simulink model "MBS_FlexibleBoom_Inverse_Dynamics"  (R2020b)
settings: Solver=ode23t  StartTime=0  StopTime=17  FixedStep=.00001  MaxStep=1e-3  RelTol=1e-3
model workspace: external: MATLAB File C:\GitHub\UiA_GreenCrane_TestBed\Simulation Models\Crane\Rigid - MBS model\param_MBS_FlexibleBoom_Inverse_Dynamics.m (data not in the file)
values from neighbouring files (symbols this model uses):
  d_eff_long = sqrt(2*J_sec_long*k_eff_long)    [param_MBS_FlexibleBoom_Inverse_Dynamics.m]
  d_eff_short = sqrt(2*J_sec_short*k_eff_short)    [param_MBS_FlexibleBoom_Inverse_Dynamics.m]
  DR = 1    [param_MBS_FlexibleBoom_Inverse_Dynamics.m]
  k_eff_long = E*I/I_sec_long    (= 3050381.94041)    [param_MBS_FlexibleBoom_Inverse_Dynamics.m]
  k_eff_short = E*I/I_sec_short    (= 13451432.5427)    [param_MBS_FlexibleBoom_Inverse_Dynamics.m]
  KR = 1    [param_MBS_FlexibleBoom_Inverse_Dynamics.m]
  v_cyl_0 = 0.0    (= 0)    [param_MBS_FlexibleBoom_Inverse_Dynamics.m]
  x_cyl_0 = 0.05    [param_MBS_FlexibleBoom_Inverse_Dynamics.m]
undefined symbols (not defined in the file or in its folder): smiData, X, Y, Z
libraries: sm_lib x190, nesl_utility x26
(part 1 of 5)
settings Model: Creator=Zygis  LastModifiedBy=danielh
settings SolverCC: ZeroCrossAlgorithm=Adaptive
settings DataIOCC: ExternalInput=getinputstruct(report1)  InitialState=getstatestruct(report1)  ReturnWorkspaceOutputs=off  Refine=2
settings DebuggingCC: IgnoredZcDiagnostic=none  UniqueDataStoreMsg=error  UnderSpecifiedDimensionMsg=warning  ArithmeticOperatorsInVariantConditions=warning
settings HardwareCC: TargetBitPerPointer=64  TargetBitPerSizeT=64  TargetBitPerPtrDiffT=64  TargetLongLongMode=on  TargetIntDivRoundTo=Zero  TargetEndianess=LittleEndian  TargetWordSize=64  TargetHWDeviceType=MATLAB Host  ProdEqTarget=off
settings SFSimCC: SimUseLocalCustomCode=off  CustomCodeUndefinedFunction=UseInterfaceOnly
settings RTWCC: Description=Rapid Simulation Target  SystemTargetFile=rsim.tlc  TemplateMakefile=rsim_default_tmf  GenerateReport=on  RTWUseLocalCustomCode=off
settings RSimTargetCC: TargetLangStandard=C99 (ISO)
settings DiagnosticsConfigSet: SimMechanicsJointTargetOverSpecification=warning

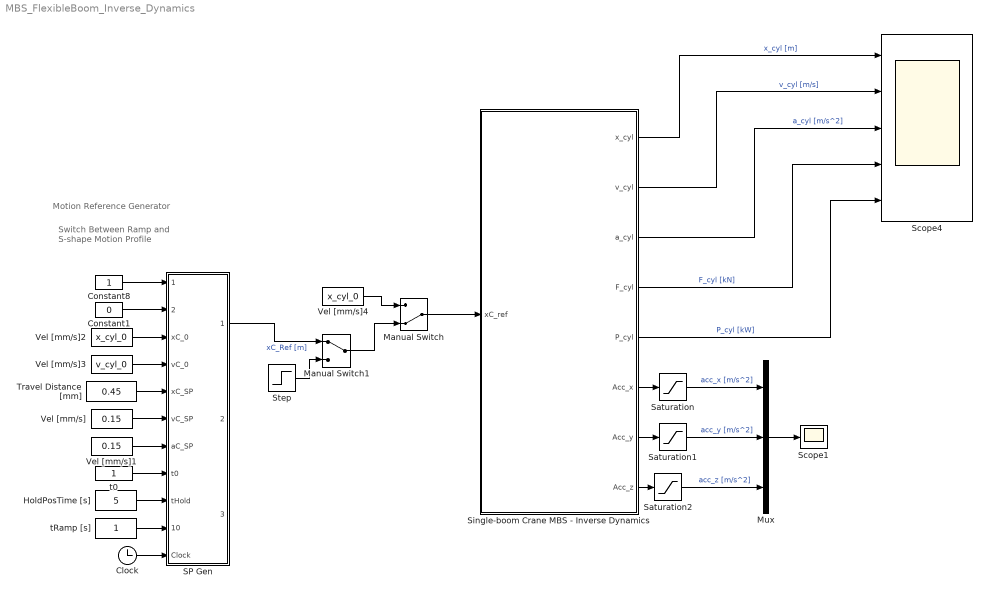
== system MBS_FlexibleBoom_Inverse_Dynamics ==
  note: Motion Reference Generator
  note: Switch Between
      | Ramp and S-shape
      | Motion Profile
  Clock : Clock
  Constant1 : Constant  Value=0  OutDataTypeStr=boolean
  Constant8 : Constant  OutDataTypeStr=boolean
  HoldPosTime [s] : Constant  Value=5
  Manual Switch : ManualSwitch  CurrentSetting=0
  Manual Switch1 : ManualSwitch
  Mux : Mux  Inputs=3
  SP Gen : Subsystem
  Saturation : Saturate  UpperLimit=2  LowerLimit=-2
  Saturation1 : Saturate  UpperLimit=2  LowerLimit=-2
  Saturation2 : Saturate  UpperLimit=2  LowerLimit=-2
  Scope1 : Scope
  Scope4 : Scope  NumInputPorts=5
  Single-boom Crane MBS - Inverse Dynamics : Subsystem  VariantControl=Flexible_model
  Step : Step  Before=x_cyl_0  After=0.1  SampleTime=0
  Travel Distance [mm] : Constant  Value=0.45
  Vel [mm/s] : Constant  Value=0.15
  Vel [mm/s]1 : Constant  Value=0.15
  Vel [mm/s]2 : Constant  Value=x_cyl_0
  Vel [mm/s]3 : Constant  Value=v_cyl_0
  Vel [mm/s]4 : Constant  Value=x_cyl_0
  t0 : Constant
  tRamp [s] : Constant
  wires:
  Single-boom Crane MBS - Inverse Dynamics/1(x_cyl) -> Scope4/1  "x_cyl [m]"
  Single-boom Crane MBS - Inverse Dynamics/2(v_cyl) -> Scope4/2  "v_cyl [m/s]"
  Manual Switch/1 -> Single-boom Crane MBS - Inverse Dynamics/1(xC_ref)
  Single-boom Crane MBS - Inverse Dynamics/3(a_cyl) -> Scope4/3  "a_cyl [m/s^2]"
  Single-boom Crane MBS - Inverse Dynamics/4(F_cyl) -> Scope4/4  "F_cyl [kN]"
  Vel [mm/s]3/1 -> SP Gen/4(vC_0)
  t0/1 -> SP Gen/8(t0)
  Constant8/1 -> SP Gen/1(Enable)
  Clock/1 -> SP Gen/11(Clock)
  Vel [mm/s]2/1 -> SP Gen/3(xC_0)
  Vel [mm/s]/1 -> SP Gen/6(vC_SP)
  Constant1/1 -> SP Gen/2(S-shape On)
  Travel Distance [mm]/1 -> SP Gen/5(xC_SP)
  tRamp [s]/1 -> SP Gen/10(tRamp)
  HoldPosTime [s]/1 -> SP Gen/9(tHold)
  Vel [mm/s]1/1 -> SP Gen/7(aC_SP)
  SP Gen/1(xC_ref) -> Manual Switch1/1  "xC_Ref [m]"
  Single-boom Crane MBS - Inverse Dynamics/5(P_cyl) -> Scope4/5  "P_cyl [kW]"
  Vel [mm/s]4/1 -> Manual Switch/1
  Step/1 -> Manual Switch1/2
  Manual Switch1/1 -> Manual Switch/2
  Single-boom Crane MBS - Inverse Dynamics/6(Acc_x) -> Saturation/1
  Single-boom Crane MBS - Inverse Dynamics/7(Acc_y) -> Saturation1/1
  Single-boom Crane MBS - Inverse Dynamics/8(Acc_z) -> Saturation2/1
  Mux/1 -> Scope1/1
  Saturation/1 -> Mux/1  "acc_x [m/s^2]"
  Saturation1/1 -> Mux/2  "acc_y [m/s^2]"
  Saturation2/1 -> Mux/3  "acc_z [m/s^2]"

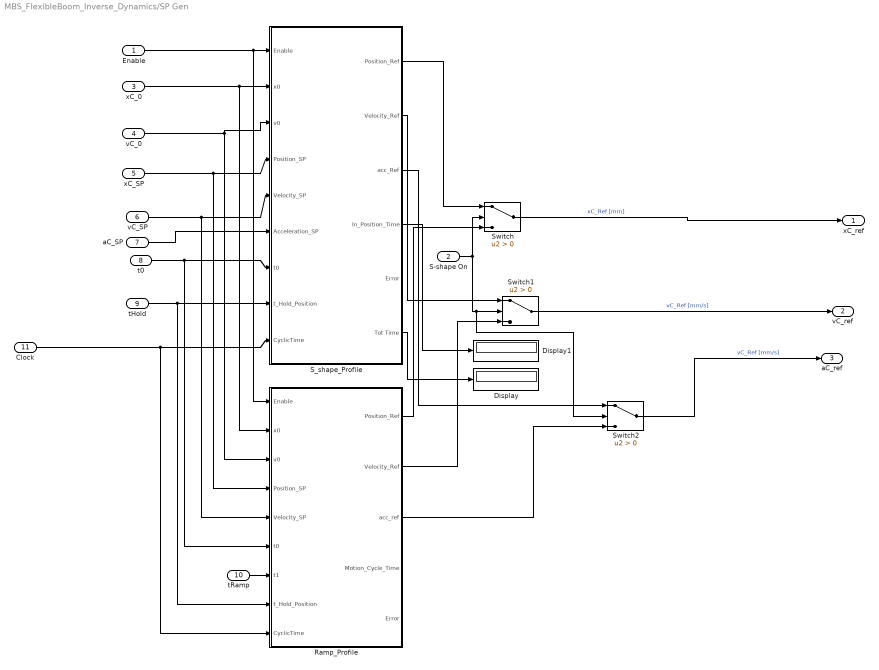
== system MBS_FlexibleBoom_Inverse_Dynamics/SP Gen ==
  Enable : Inport
  S-shape On : Inport  Port=2
  xC_0 : Inport  Port=3
  vC_0 : Inport  Port=4
  xC_SP : Inport  Port=5
  vC_SP : Inport  Port=6
  aC_SP : Inport  Port=7
  t0 : Inport  Port=8
  tHold : Inport  Port=9
  tRamp : Inport  Port=10
  Clock : Inport  Port=11
  Display : Display
  Display1 : Display
  Ramp_Profile : Subsystem  TreatAsAtomicUnit=on  VariantControl=Ramp_Profile
  S_shape_Profile : Subsystem  VariantControl=S_shape_Profile
  Switch : Switch  Criteria=u2 > Threshold
  Switch1 : Switch  Criteria=u2 > Threshold
  Switch2 : Switch  Criteria=u2 > Threshold
  xC_ref : Outport  VectorParamsAs1DForOutWhenUnconnected=off
  vC_ref : Outport  Port=2  VectorParamsAs1DForOutWhenUnconnected=off
  aC_ref : Outport  Port=3  VectorParamsAs1DForOutWhenUnconnected=off
  wires:
  t0/1 -> Ramp_Profile/6(t0), S_shape_Profile/7(t0)
  vC_SP/1 -> Ramp_Profile/5(Velocity_SP), S_shape_Profile/5(Velocity_SP)
  xC_0/1 -> Ramp_Profile/2(x0), S_shape_Profile/2(x0)
  xC_SP/1 -> Ramp_Profile/4(Position_SP), S_shape_Profile/4(Position_SP)
  Enable/1 -> Ramp_Profile/1(Enable), S_shape_Profile/1(Enable)
  tHold/1 -> Ramp_Profile/8(t_Hold_Position), S_shape_Profile/8(t_Hold_Position)
  S_shape_Profile/1(Position_Ref) -> Switch/1
  Ramp_Profile/1(Position_Ref) -> Switch/3
  S_shape_Profile/2(Velocity_Ref) -> Switch1/1
  S-shape On/1 -> Switch/2, Switch2/2, Switch1/2
  tRamp/1 -> Ramp_Profile/7(t1)
  S_shape_Profile/6(Tot Time) -> Display/1
  S_shape_Profile/4(" In_Position_Time") -> Display1/1
  vC_0/1 -> S_shape_Profile/3(v0), Ramp_Profile/3(v0)
  aC_SP/1 -> S_shape_Profile/6(Acceleration_SP)
  Clock/1 -> Ramp_Profile/9(CyclicTime), S_shape_Profile/9(CyclicTime)
  Switch/1 -> xC_ref/1  "xC_Ref [mm]"
  Switch1/1 -> vC_ref/1  "vC_Ref [mm/s]"
  Ramp_Profile/2(Velocity_Ref) -> Switch1/3
  Switch2/1 -> aC_ref/1  "vC_Ref [mm/s]"
  S_shape_Profile/3(acc_Ref) -> Switch2/1
  Ramp_Profile/3(acc_ref) -> Switch2/3

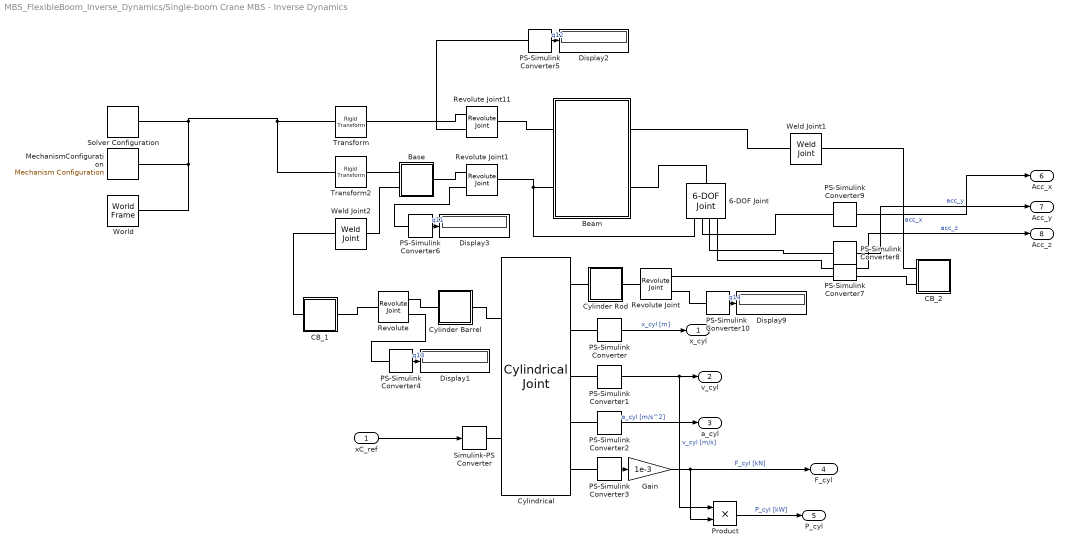
== system MBS_FlexibleBoom_Inverse_Dynamics/Single-boom Crane MBS - Inverse Dynamics ==
  xC_ref : Inport
  6-DOF Joint : sm_lib/Joints/6-DOF Joint  JointMode=Normal  SenseConstraintForce=off  SenseConstraintForceX=off  SenseConstraintForceY=off  SenseConstraintForceZ=off  SenseConstraintTorque=off  SenseConstraintTorqueX=off  SenseConstraintTorqueY=off  SenseConstraintTorqueZ=off  SenseTotalForce=off  SenseTotalForceX=off  SenseTotalForceY=off  SenseTotalForceZ=off  SenseTotalTorque=off  SenseTotalTorqueX=off  SenseTotalTorqueY=off  SenseTotalTorqueZ=off  CompositeWrenchDir=FollowerOnBase  CompositeWrenchFrame=BaseFrame  PxEquilibriumPosition=0  PxEquilibriumPositionUnits=m  PxSpringStiffness=0  PxSpringStiffnessUnits=N/m  PxDampingCoefficient=0  PxDampingCoefficientUnits=N/(m/s)  PxTorqueActuationMode=NoTorque  PxMotionActuationMode=ComputedMotion  PxSensePosition=off  PxSenseVelocity=off  PxSenseAcceleration=on  PxSenseTorqueForce=off  PxSenseLowerLimitTorqueForce=off  PxSenseUpperLimitTorqueForce=off  PxLowerLimitSpecify=off  PxLowerLimitBound=-1  PxLowerLimitBoundUnits=m  PxLowerLimitStiffness=1e6  PxLowerLimitStiffnessUnits=N/m  PxLowerLimitDamping=1e3  PxLowerLimitDampingUnits=N/(m/s)  PxLowerLimitTransitionRegionWidth=1e-4  PxLowerLimitTransitionRegionWidthUnits=m  PxUpperLimitSpecify=off  PxUpperLimitBound=1  PxUpperLimitBoundUnits=m  PxUpperLimitStiffness=1e6  PxUpperLimitStiffnessUnits=N/m  PxUpperLimitDamping=1e3  PxUpperLimitDampingUnits=N/(m/s)  PxUpperLimitTransitionRegionWidth=1e-4  PxUpperLimitTransitionRegionWidthUnits=m  PxPositionTargetSpecify=off  PxPositionTargetPriority=High  PxPositionTargetValue=0  PxPositionTargetValueUnits=m  PxVelocityTargetSpecify=off  PxVelocityTargetPriority=High  PxVelocityTargetValue=0  PxVelocityTargetValueUnits=m/s  PyEquilibriumPosition=0  PyEquilibriumPositionUnits=m  PySpringStiffness=0  PySpringStiffnessUnits=N/m  PyDampingCoefficient=0  PyDampingCoefficientUnits=N/(m/s)  PyTorqueActuationMode=NoTorque  PyMotionActuationMode=ComputedMotion  PySensePosition=off  PySenseVelocity=off  PySenseAcceleration=on  PySenseTorqueForce=off  PySenseLowerLimitTorqueForce=off  PySenseUpperLimitTorqueForce=off  PyLowerLimitSpecify=off  PyLowerLimitBound=-1  PyLowerLimitBoundUnits=m  PyLowerLimitStiffness=1e6  PyLowerLimitStiffnessUnits=N/m  PyLowerLimitDamping=1e3  PyLowerLimitDampingUnits=N/(m/s)  PyLowerLimitTransitionRegionWidth=1e-4  PyLowerLimitTransitionRegionWidthUnits=m  PyUpperLimitSpecify=off  PyUpperLimitBound=1  PyUpperLimitBoundUnits=m  PyUpperLimitStiffness=1e6  PyUpperLimitStiffnessUnits=N/m  PyUpperLimitDamping=1e3  PyUpperLimitDampingUnits=N/(m/s)  PyUpperLimitTransitionRegionWidth=1e-4  PyUpperLimitTransitionRegionWidthUnits=m  PyPositionTargetSpecify=off  PyPositionTargetPriority=High  PyPositionTargetValue=0  PyPositionTargetValueUnits=m  PyVelocityTargetSpecify=off  PyVelocityTargetPriority=High  PyVelocityTargetValue=0  PyVelocityTargetValueUnits=m/s  PzEquilibriumPosition=0  PzEquilibriumPositionUnits=m  PzSpringStiffness=0  PzSpringStiffnessUnits=N/m  PzDampingCoefficient=0  PzDampingCoefficientUnits=N/(m/s)  PzTorqueActuationMode=NoTorque  PzMotionActuationMode=ComputedMotion  PzSensePosition=off  PzSenseVelocity=off  PzSenseAcceleration=on  PzSenseTorqueForce=off  PzSenseLowerLimitTorqueForce=off  PzSenseUpperLimitTorqueForce=off  PzLowerLimitSpecify=off  PzLowerLimitBound=-1  PzLowerLimitBoundUnits=m  PzLowerLimitStiffness=1e6  PzLowerLimitStiffnessUnits=N/m  PzLowerLimitDamping=1e3  PzLowerLimitDampingUnits=N/(m/s)  PzLowerLimitTransitionRegionWidth=1e-4  PzLowerLimitTransitionRegionWidthUnits=m  PzUpperLimitSpecify=off  PzUpperLimitBound=1  PzUpperLimitBoundUnits=m  PzUpperLimitStiffness=1e6  PzUpperLimitStiffnessUnits=N/m  PzUpperLimitDamping=1e3  PzUpperLimitDampingUnits=N/(m/s)  PzUpperLimitTransitionRegionWidth=1e-4  PzUpperLimitTransitionRegionWidthUnits=m  PzPositionTargetSpecify=off  PzPositionTargetPriority=High  PzPositionTargetValue=0  PzPositionTargetValueUnits=m  PzVelocityTargetSpecify=off  PzVelocityTargetPriority=High  PzVelocityTargetValue=0  PzVelocityTargetValueUnits=m/s  SphDefPosRotationMethod=None  SphDefPosRotationAngleUnits=deg  SphDefPosRotationStandardAxis=+Z  SphDefPosRotationAngle=0.0  SphDefPosRotationArbitraryAxis=[0 0 1]  SphDefPosFollAlignAxisA=+X  SphDefPosBaseAlignAxisA=+Y  SphDefPosFollAlignAxisB=+Y  SphDefPosBaseAlignAxisB=+Z  SphDefPosRotationSequenceAxes=FollowerAxes  SphDefPosRotationSequence=XYX  SphDefPosRotationSequenceAngles=[0 0 0]  SphDefPosRotationSequenceAnglesUnits=deg  SphDefPosRotationMatrix=[1 0 0; 0 1 0; 0 0 1]  SphEqPosRotationMethod=None  SphEqPosRotationAngleUnits=deg  SphEqPosRotationStandardAxis=+Z  SphEqPosRotationAngle=0.0  SphEqPosRotationArbitraryAxis=[0 0 1]  SphEqPosFollAlignAxisA=+X  SphEqPosBaseAlignAxisA=+Y  SphEqPosFollAlignAxisB=+Y  SphEqPosBaseAlignAxisB=+Z  SphEqPosRotationSequenceAxes=FollowerAxes  SphEqPosRotationSequence=XYX  SphEqPosRotationSequenceAngles=[0 0 0]  SphEqPosRotationSequenceAnglesUnits=deg  SphEqPosRotationMatrix=[1 0 0; 0 1 0; 0 0 1]  SphSpringStiffness=0  SphSpringStiffnessUnits=N*m/deg  SphDampingCoefficient=0  SphDampingCoefficientUnits=N*m/(deg/s)  SphActuateTorqueX=off  SphActuateTorqueY=off  SphActuateTorqueZ=off  SphActuateTorque=off  SphTorqueActuationMode=NoTorque  SphMotionActuationMode=ComputedMotion  SphActuationFrame=BaseFrame  SphSensePosition=off  SphSenseVelocityX=off  SphSenseVelocityY=off  SphSenseVelocityZ=off  SphSenseVelocity=off  SphSenseAccelerationX=off  SphSenseAccelerationY=off  SphSenseAccelerationZ=off  SphSenseAcceleration=off  SphSenseTorqueX=off  SphSenseTorqueY=off  SphSenseTorqueZ=off  SphSenseTorqueForce=off  SphSenseLowerLimitTorqueMag=off  SphSenseUpperLimitTorqueMag=off  SphSensingFrame=BaseFrame  SphLowerLimitSpecify=off  SphLowerLimitBound=15  SphLowerLimitBoundUnits=deg  SphLowerLimitStiffness=1e4  SphLowerLimitStiffnessUnits=N*m/deg  SphLowerLimitDamping=10  SphLowerLimitDampingUnits=N*m/(deg/s)  SphLowerLimitTransitionRegionWidth=0.1  SphLowerLimitTransitionRegionWidthUnits=deg  SphUpperLimitSpecify=off  SphUpperLimitBound=45  SphUpperLimitBoundUnits=deg  SphUpperLimitStiffness=1e4  SphUpperLimitStiffnessUnits=N*m/deg  SphUpperLimitDamping=10  SphUpperLimitDampingUnits=N*m/(deg/s)  SphUpperLimitTransitionRegionWidth=0.1  SphUpperLimitTransitionRegionWidthUnits=deg  SphPositionTargetRotationMethod=None  SphPositionTargetRotationAngleUnits=deg  SphPositionTargetRotationStandardAxis=+Z  SphPositionTargetRotationAngle=0.0  SphPositionTargetRotationArbitraryAxis=[0 0 1]  SphPositionTargetFollAlignAxisA=+X  SphPositionTargetBaseAlignAxisA=+Y  SphPositionTargetFollAlignAxisB=+Y  SphPositionTargetBaseAlignAxisB=+Z  SphPositionTargetRotationSequenceAxes=FollowerAxes  SphPositionTargetRotationSequence=XYX  SphPositionTargetRotationSequenceAngles=[0 0 0]  SphPositionTargetRotationSequenceAnglesUnits=deg  SphPositionTargetRotationMatrix=[1 0 0; 0 1 0; 0 0 1]  SphPositionTargetSpecify=off  SphPositionTargetPriority=High  SphVelocityTargetValue=[0 0 0]  SphVelocityTargetValueUnits=deg/s  SphVelocityTargetSpecify=off  SphVelocityTargetPriority=High  SphVelocityTargetInFollowerFrame=on
  Base : Subsystem
  Beam : Subsystem
  CB_1 : Subsystem
  CB_2 : Subsystem
  Cylinder Barrel : Subsystem
  Cylinder Rod : Subsystem
  Cylindrical : sm_lib/Joints/Cylindrical Joint  JointMode=Normal  SenseConstraintForce=off  SenseConstraintForceX=off  SenseConstraintForceY=off  SenseConstraintForceZ=off  SenseConstraintTorque=off  SenseConstraintTorqueX=off  SenseConstraintTorqueY=off  SenseConstraintTorqueZ=off  SenseTotalForce=off  SenseTotalForceX=off  SenseTotalForceY=off  SenseTotalForceZ=off  SenseTotalTorque=off  SenseTotalTorqueX=off  SenseTotalTorqueY=off  SenseTotalTorqueZ=off  CompositeWrenchDir=FollowerOnBase  CompositeWrenchFrame=BaseFrame  PzEquilibriumPosition=0  PzEquilibriumPositionUnits=m  PzSpringStiffness=0  PzSpringStiffnessUnits=N/m  PzDampingCoefficient=0  PzDampingCoefficientUnits=N/(m/s)  PzTorqueActuationMode=ComputedTorque  PzMotionActuationMode=InputMotion  PzSensePosition=on  PzSenseVelocity=on  PzSenseAcceleration=on  PzSenseTorqueForce=on  PzSenseLowerLimitTorqueForce=off  PzSenseUpperLimitTorqueForce=off  PzLowerLimitSpecify=off  PzLowerLimitBound=-1  PzLowerLimitBoundUnits=m  PzLowerLimitStiffness=1e6  PzLowerLimitStiffnessUnits=N/m  PzLowerLimitDamping=1e3  PzLowerLimitDampingUnits=N/(m/s)  PzLowerLimitTransitionRegionWidth=1e-4  PzLowerLimitTransitionRegionWidthUnits=m  PzUpperLimitSpecify=off  PzUpperLimitBound=1  PzUpperLimitBoundUnits=m  PzUpperLimitStiffness=1e6  PzUpperLimitStiffnessUnits=N/m  PzUpperLimitDamping=1e3  PzUpperLimitDampingUnits=N/(m/s)  PzUpperLimitTransitionRegionWidth=1e-4  PzUpperLimitTransitionRegionWidthUnits=m  PzPositionTargetSpecify=on  PzPositionTargetPriority=High  PzPositionTargetValue=x_cyl_0  PzPositionTargetValueUnits=m  PzVelocityTargetSpecify=on  PzVelocityTargetPriority=High  PzVelocityTargetValue=v_cyl_0  PzVelocityTargetValueUnits=m/s  RzEquilibriumPosition=0  RzEquilibriumPositionUnits=rad  RzSpringStiffness=0  RzSpringStiffnessUnits=N*m/rad  RzDampingCoefficient=0  RzDampingCoefficientUnits=N*m/(rad/s)  RzTorqueActuationMode=NoTorque  RzMotionActuationMode=ComputedMotion  RzSensePosition=off  RzSenseVelocity=off  RzSenseAcceleration=off  RzSenseTorqueForce=off  RzSenseLowerLimitTorqueForce=off  RzSenseUpperLimitTorqueForce=off  RzLowerLimitSpecify=off  RzLowerLimitBound=-90  RzLowerLimitBoundUnits=deg  RzLowerLimitStiffness=1e4  RzLowerLimitStiffnessUnits=N*m/deg  RzLowerLimitDamping=10  RzLowerLimitDampingUnits=N*m/(deg/s)  RzLowerLimitTransitionRegionWidth=0.1  RzLowerLimitTransitionRegionWidthUnits=deg  RzUpperLimitSpecify=off  RzUpperLimitBound=90  RzUpperLimitBoundUnits=deg  RzUpperLimitStiffness=1e4  RzUpperLimitStiffnessUnits=N*m/deg  RzUpperLimitDamping=10  RzUpperLimitDampingUnits=N*m/(deg/s)  RzUpperLimitTransitionRegionWidth=0.1  RzUpperLimitTransitionRegionWidthUnits=deg  RzPositionTargetSpecify=on  RzPositionTargetPriority=High  RzPositionTargetValue=q15  RzPositionTargetValueUnits=rad  RzVelocityTargetSpecify=off  RzVelocityTargetPriority=High  RzVelocityTargetValue=0  RzVelocityTargetValueUnits=rad/s
  Display{1..3,9} (4 alike) : Display
  Gain : Gain  Gain=1e-3
  MechanismConfiguration : sm_lib/Utilities/Mechanism Configuration  UniformGravity=Constant  GravityVector=[0 -9.80665 0]  GravityVectorUnits=m/s^2  GravityUnits=m/s^2  LinearizationDelta=0.001  JointModeTransitionNonlinearIterations=2
  PS-Simulink Converter{,1..10} (11 alike) : nesl_utility/PS-Simulink Converter  PhysicalDomain=network_engine_domain  SubClassName=ps_output  LeftPortType=input  RightPortType=output  PseudoPeriodic=off  Frequencies=[]  Unit=1  AffineConversion=off
  Product : Product
  Revolute : sm_lib/Joints/Revolute Joint  JointMode=Normal  SenseConstraintForce=off  SenseConstraintForceX=off  SenseConstraintForceY=off  SenseConstraintForceZ=off  SenseConstraintTorque=off  SenseConstraintTorqueX=off  SenseConstraintTorqueY=off  SenseConstraintTorqueZ=off  SenseTotalForce=off  SenseTotalForceX=off  SenseTotalForceY=off  SenseTotalForceZ=off  SenseTotalTorque=off  SenseTotalTorqueX=off  SenseTotalTorqueY=off  SenseTotalTorqueZ=off  CompositeWrenchDir=FollowerOnBase  CompositeWrenchFrame=BaseFrame  EquilibriumPosition=0  EquilibriumPositionUnits=rad  SpringStiffness=0  SpringStiffnessUnits=N*m/rad  DampingCoefficient=0  DampingCoefficientUnits=N*m/(rad/s)  TorqueActuationMode=NoTorque  MotionActuationMode=ComputedMotion  SensePosition=on  SenseVelocity=off  SenseAcceleration=off  SenseTorqueForce=off  SenseLowerLimitTorqueForce=off  SenseUpperLimitTorqueForce=off  LowerLimitSpecify=off  LowerLimitBound=-90  LowerLimitBoundUnits=deg  LowerLimitStiffness=1e4  LowerLimitStiffnessUnits=N*m/deg  LowerLimitDamping=10  LowerLimitDampingUnits=N*m/(deg/s)  LowerLimitTransitionRegionWidth=0.1  LowerLimitTransitionRegionWidthUnits=deg  UpperLimitSpecify=off  UpperLimitBound=90  UpperLimitBoundUnits=deg  UpperLimitStiffness=1e4  UpperLimitStiffnessUnits=N*m/deg  UpperLimitDamping=10  UpperLimitDampingUnits=N*m/(deg/s)  UpperLimitTransitionRegionWidth=0.1  UpperLimitTransitionRegionWidthUnits=deg  PositionTargetSpecify=on  PositionTargetPriority=High  PositionTargetValue=q13  PositionTargetValueUnits=rad  VelocityTargetSpecify=on  VelocityTargetPriority=High  VelocityTargetValue=0  VelocityTargetValueUnits=rad/s
  Revolute Joint : sm_lib/Joints/Revolute Joint  JointMode=Normal  SenseConstraintForce=off  SenseConstraintForceX=off  SenseConstraintForceY=off  SenseConstraintForceZ=off  SenseConstraintTorque=off  SenseConstraintTorqueX=off  SenseConstraintTorqueY=off  SenseConstraintTorqueZ=off  SenseTotalForce=off  SenseTotalForceX=off  SenseTotalForceY=off  SenseTotalForceZ=off  SenseTotalTorque=off  SenseTotalTorqueX=off  SenseTotalTorqueY=off  SenseTotalTorqueZ=off  CompositeWrenchDir=FollowerOnBase  CompositeWrenchFrame=BaseFrame  EquilibriumPosition=0  EquilibriumPositionUnits=deg  SpringStiffness=0  SpringStiffnessUnits=N*m/deg  DampingCoefficient=0  DampingCoefficientUnits=N*m/(deg/s)  TorqueActuationMode=NoTorque  MotionActuationMode=ComputedMotion  SensePosition=on  SenseVelocity=off  SenseAcceleration=off  SenseTorqueForce=off  SenseLowerLimitTorqueForce=off  SenseUpperLimitTorqueForce=off  LowerLimitSpecify=off  LowerLimitBound=-90  LowerLimitBoundUnits=deg  LowerLimitStiffness=1e4  LowerLimitStiffnessUnits=N*m/deg  LowerLimitDamping=10  LowerLimitDampingUnits=N*m/(deg/s)  LowerLimitTransitionRegionWidth=0.1  LowerLimitTransitionRegionWidthUnits=deg  UpperLimitSpecify=off  UpperLimitBound=90  UpperLimitBoundUnits=deg  UpperLimitStiffness=1e4  UpperLimitStiffnessUnits=N*m/deg  UpperLimitDamping=10  UpperLimitDampingUnits=N*m/(deg/s)  UpperLimitTransitionRegionWidth=0.1  UpperLimitTransitionRegionWidthUnits=deg  PositionTargetSpecify=on  PositionTargetPriority=High  PositionTargetValue=q14  PositionTargetValueUnits=rad  VelocityTargetSpecify=on  VelocityTargetPriority=High  VelocityTargetValue=0  VelocityTargetValueUnits=rad/s
  Revolute Joint1 : sm_lib/Joints/Revolute Joint  JointMode=Normal  SenseConstraintForce=off  SenseConstraintForceX=off  SenseConstraintForceY=off  SenseConstraintForceZ=off  SenseConstraintTorque=off  SenseConstraintTorqueX=off  SenseConstraintTorqueY=off  SenseConstraintTorqueZ=off  SenseTotalForce=off  SenseTotalForceX=off  SenseTotalForceY=off  SenseTotalForceZ=off  SenseTotalTorque=off  SenseTotalTorqueX=off  SenseTotalTorqueY=off  SenseTotalTorqueZ=off  CompositeWrenchDir=FollowerOnBase  CompositeWrenchFrame=BaseFrame  EquilibriumPosition=0  EquilibriumPositionUnits=deg  SpringStiffness=0  SpringStiffnessUnits=N*m/deg  DampingCoefficient=0  DampingCoefficientUnits=N*m/(deg/s)  TorqueActuationMode=NoTorque  MotionActuationMode=ComputedMotion  SensePosition=on  SenseVelocity=off  SenseAcceleration=off  SenseTorqueForce=off  SenseLowerLimitTorqueForce=off  SenseUpperLimitTorqueForce=off  LowerLimitSpecify=off  LowerLimitBound=-90  LowerLimitBoundUnits=deg  LowerLimitStiffness=1e4  LowerLimitStiffnessUnits=N*m/deg  LowerLimitDamping=10  LowerLimitDampingUnits=N*m/(deg/s)  LowerLimitTransitionRegionWidth=0.1  LowerLimitTransitionRegionWidthUnits=deg  UpperLimitSpecify=off  UpperLimitBound=90  UpperLimitBoundUnits=deg  UpperLimitStiffness=1e4  UpperLimitStiffnessUnits=N*m/deg  UpperLimitDamping=10  UpperLimitDampingUnits=N*m/(deg/s)  UpperLimitTransitionRegionWidth=0.1  UpperLimitTransitionRegionWidthUnits=deg  PositionTargetSpecify=on  PositionTargetPriority=High  PositionTargetValue=q11  PositionTargetValueUnits=rad  VelocityTargetSpecify=on  VelocityTargetPriority=High  VelocityTargetValue=0  VelocityTargetValueUnits=rad/s
  Revolute Joint11 : sm_lib/Joints/Revolute Joint  JointMode=Normal  SenseConstraintForce=off  SenseConstraintForceX=off  SenseConstraintForceY=off  SenseConstraintForceZ=off  SenseConstraintTorque=off  SenseConstraintTorqueX=off  SenseConstraintTorqueY=off  SenseConstraintTorqueZ=off  SenseTotalForce=off  SenseTotalForceX=off  SenseTotalForceY=off  SenseTotalForceZ=off  SenseTotalTorque=off  SenseTotalTorqueX=off  SenseTotalTorqueY=off  SenseTotalTorqueZ=off  CompositeWrenchDir=FollowerOnBase  CompositeWrenchFrame=BaseFrame  EquilibriumPosition=0  EquilibriumPositionUnits=deg  SpringStiffness=0  SpringStiffnessUnits=N*m/deg  DampingCoefficient=0  DampingCoefficientUnits=N*m/(deg/s)  TorqueActuationMode=NoTorque  MotionActuationMode=ComputedMotion  SensePosition=on  SenseVelocity=off  SenseAcceleration=off  SenseTorqueForce=off  SenseLowerLimitTorqueForce=off  SenseUpperLimitTorqueForce=off  LowerLimitSpecify=off  LowerLimitBound=-90  LowerLimitBoundUnits=deg  LowerLimitStiffness=1e4  LowerLimitStiffnessUnits=N*m/deg  LowerLimitDamping=10  LowerLimitDampingUnits=N*m/(deg/s)  LowerLimitTransitionRegionWidth=0.1  LowerLimitTransitionRegionWidthUnits=deg  UpperLimitSpecify=off  UpperLimitBound=90  UpperLimitBoundUnits=deg  UpperLimitStiffness=1e4  UpperLimitStiffnessUnits=N*m/deg  UpperLimitDamping=10  UpperLimitDampingUnits=N*m/(deg/s)  UpperLimitTransitionRegionWidth=0.1  UpperLimitTransitionRegionWidthUnits=deg  PositionTargetSpecify=on  PositionTargetPriority=High  PositionTargetValue=q12  PositionTargetValueUnits=rad  VelocityTargetSpecify=on  VelocityTargetPriority=High  VelocityTargetValue=0  VelocityTargetValueUnits=rad/s
  Simulink-PS Converter : nesl_utility/Simulink-PS Converter  PhysicalDomain=network_engine_domain  SubClassName=ps_input  LeftPortType=input  RightPortType=output  PseudoPeriodic=off  Frequencies=[]  NoiseDistribution=none  NoiseParameters=[]  Unit=1  AffineConversion=off  FilteringAndDerivatives=filter  SimscapeFilterOrder=2  InputFilterTimeConstant=0.001  UdotUserProvided=0
  Solver Configuration : nesl_utility/Solver Configuration  PhysicalDomain=network_engine_domain  SubClassName=solver  LeftPortType=input  RightPortType=generic  Tones=[]  Harmonics=[]  SimulateNoise=off  Profile=off  UseLocalSampling=off  EnableSwitchedLinearOptims=on  FrequencyDomain=off  UseCCode=off  RelTol=0.001  AbsTol=1e-06  MinStep=1e-09  ToWorkspace=off  RevertToSquareIcSolve=off  NumHomotopyIterations=100  PhasorMode=off  PhasorModeNumHarmonics=1  DoDC=on  ResidualTolerance=1e-09  UseLocalSolver=off  LocalSolverChoice=NE_BACKWARD_EULER_ADVANCER  LocalSolverSampleTime=0.001  DoFixedCost=off  MaxNonlinIter=3  MaxModeIter=2  ComputeImpulses=off  ImpulseIterations=2  LinearAlgebra=Sparse  EquationFormulation=NE_TIME_EF  DelaysMemoryBudget=1024  AutomaticFiltering=off  FilteringTimeConstant=0.001  PartitionStorageMethod=AS_NEEDED  PartitionMemoryBudget=1024  PartitionMethod=FAST
  Transform : sm_lib/Frames and Transforms/Rigid Transform  TranslationMethod=Cartesian  TranslationStandardOffset=0  TranslationLengthUnit=mm  TranslationStandardAxis=+Z  TranslationCartesianOffset=smiData.RigidTransform(8).translation  TranslationROffset=0  TranslationROffsetUnits=m  TranslationZOffset=0  TranslationZOffsetUnits=m  TranslationThetaOffset=0  TranslationThetaOffsetUnits=deg  RotationMethod=ArbitraryAxis  RotationAngleUnits=rad  RotationStandardAxis=+Z  RotationAngle=smiData.RigidTransform(8).angle  RotationArbitraryAxis=smiData.RigidTransform(8).axis  FollAlignAxisA=+X  BaseAlignAxisA=+Y  FollAlignAxisB=+Y  BaseAlignAxisB=+Z  RotationSequenceAxes=FollowerAxes  RotationSequence=XYX  RotationSequenceAngles=[0 0 0]  RotationSequenceAnglesUnits=deg  RotationMatrix=[1 0 0; 0 1 0; 0 0 1]
  Transform2 : sm_lib/Frames and Transforms/Rigid Transform  TranslationMethod=Cartesian  TranslationStandardOffset=0  TranslationLengthUnit=mm  TranslationStandardAxis=+Z  TranslationCartesianOffset=smiData.RigidTransform(12).translation  TranslationROffset=0  TranslationROffsetUnits=m  TranslationZOffset=0  TranslationZOffsetUnits=m  TranslationThetaOffset=0  TranslationThetaOffsetUnits=deg  RotationMethod=ArbitraryAxis  RotationAngleUnits=rad  RotationStandardAxis=+Z  RotationAngle=smiData.RigidTransform(12).angle  RotationArbitraryAxis=smiData.RigidTransform(12).axis  FollAlignAxisA=+X  BaseAlignAxisA=+Y  FollAlignAxisB=+Y  BaseAlignAxisB=+Z  RotationSequenceAxes=FollowerAxes  RotationSequence=XYX  RotationSequenceAngles=[0 0 0]  RotationSequenceAnglesUnits=deg  RotationMatrix=[1 0 0; 0 1 0; 0 0 1]
  Weld Joint1 : sm_lib/Joints/Weld Joint  JointMode=Normal  SenseConstraintForce=off  SenseConstraintForceX=off  SenseConstraintForceY=off  SenseConstraintForceZ=off  SenseConstraintTorque=off  SenseConstraintTorqueX=off  SenseConstraintTorqueY=off  SenseConstraintTorqueZ=off  SenseTotalForce=off  SenseTotalForceX=off  SenseTotalForceY=off  SenseTotalForceZ=off  SenseTotalTorque=off  SenseTotalTorqueX=off  SenseTotalTorqueY=off  SenseTotalTorqueZ=off  CompositeWrenchDir=FollowerOnBase  CompositeWrenchFrame=BaseFrame
  Weld Joint2 : sm_lib/Joints/Weld Joint  JointMode=Normal  SenseConstraintForce=off  SenseConstraintForceX=off  SenseConstraintForceY=off  SenseConstraintForceZ=off  SenseConstraintTorque=off  SenseConstraintTorqueX=off  SenseConstraintTorqueY=off  SenseConstraintTorqueZ=off  SenseTotalForce=off  SenseTotalForceX=off  SenseTotalForceY=off  SenseTotalForceZ=off  SenseTotalTorque=off  SenseTotalTorqueX=off  SenseTotalTorqueY=off  SenseTotalTorqueZ=off  CompositeWrenchDir=FollowerOnBase  CompositeWrenchFrame=BaseFrame
  World : sm_lib/Frames and Transforms/World Frame
  x_cyl : Outport  VectorParamsAs1DForOutWhenUnconnected=off
  v_cyl : Outport  Port=2  VectorParamsAs1DForOutWhenUnconnected=off
  a_cyl : Outport  Port=3  VectorParamsAs1DForOutWhenUnconnected=off
  F_cyl : Outport  Port=4  VectorParamsAs1DForOutWhenUnconnected=off
  P_cyl : Outport  Port=5  VectorParamsAs1DForOutWhenUnconnected=off
  Acc_x : Outport  Port=6  VectorParamsAs1DForOutWhenUnconnected=off
  Acc_y : Outport  Port=7  VectorParamsAs1DForOutWhenUnconnected=off
  Acc_z : Outport  Port=8  VectorParamsAs1DForOutWhenUnconnected=off
  wires:
  xC_ref/1 -> Simulink-PS Converter/1
  PS-Simulink Converter/1 -> x_cyl/1  "x_cyl [m]"
  PS-Simulink Converter1/1 -> Product/1, v_cyl/1  "v_cyl [m/s]"
  PS-Simulink Converter2/1 -> a_cyl/1  "a_cyl [m/s^2]"
  PS-Simulink Converter3/1 -> Gain/1
  Product/1 -> P_cyl/1  "P_cyl [kW]"
  PS-Simulink Converter10/1 -> Display9/1  "q14"
  PS-Simulink Converter4/1 -> Display1/1  "q13"
  PS-Simulink Converter5/1 -> Display2/1  "q12"
  PS-Simulink Converter6/1 -> Display3/1  "q11"
  PS-Simulink Converter9/1 -> Acc_x/1  "acc_x"
  PS-Simulink Converter8/1 -> Acc_y/1  "acc_y"
  PS-Simulink Converter7/1 -> Acc_z/1  "acc_z"
  Gain/1 -> Product/2, F_cyl/1  "F_cyl [kN]"
  connections:
  World/RConn1 -- MechanismConfiguration/RConn1 -- Transform2/LConn1 -- Transform/LConn1 -- Solver Configuration/RConn1
  Cylinder Rod/LConn1 -- Cylindrical/RConn1
  Weld Joint2/LConn1 -- Base/RConn2
  PS-Simulink Converter1/LConn1 -- Cylindrical/RConn3
  PS-Simulink Converter/LConn1 -- Cylindrical/RConn2
  Revolute Joint/LConn1 -- Cylinder Rod/RConn1
  Base/RConn1 -- Transform2/RConn1
  CB_1/RConn1 -- Revolute/LConn1
  Revolute Joint1/RConn1 -- Base/LConn1
  CB_2/LConn2 -- Revolute Joint/RConn1
  Simulink-PS Converter/RConn1 -- Cylindrical/LConn2
  Beam/LConn2 -- Revolute Joint1/LConn1 -- 6-DOF Joint/RConn1
  Revolute Joint11/LConn1 -- Beam/LConn1
  Revolute Joint11/RConn1 -- Transform/RConn1
  Weld Joint1/RConn1 -- Beam/RConn1
  Weld Joint1/LConn1 -- CB_2/LConn1
  Cylinder Barrel/RConn1 -- Cylindrical/LConn1
  Cylinder Barrel/LConn1 -- Revolute/RConn1
  CB_1/LConn1 -- Weld Joint2/RConn1
  6-DOF Joint/LConn1 -- Beam/RConn2
  Cylindrical/RConn4 -- PS-Simulink Converter2/LConn1
  PS-Simulink Converter3/LConn1 -- Cylindrical/RConn5
  PS-Simulink Converter10/LConn1 -- Revolute Joint/RConn2
  PS-Simulink Converter4/LConn1 -- Revolute/RConn2
  PS-Simulink Converter5/LConn1 -- Revolute Joint11/RConn2
  PS-Simulink Converter6/LConn1 -- Revolute Joint1/RConn2
  PS-Simulink Converter7/LConn1 -- 6-DOF Joint/RConn4
  PS-Simulink Converter8/LConn1 -- 6-DOF Joint/RConn3
  PS-Simulink Converter9/LConn1 -- 6-DOF Joint/RConn2

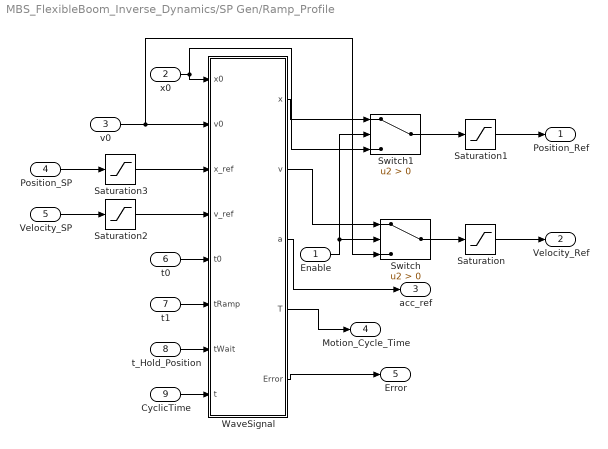
== system MBS_FlexibleBoom_Inverse_Dynamics/SP Gen/Ramp_Profile ==
  Enable : Inport  OutDataTypeStr=boolean
  x0 : Inport  Port=2
  v0 : Inport  Port=3
  Position_SP : Inport  Port=4
  Velocity_SP : Inport  Port=5
  t0 : Inport  Port=6
  t1 : Inport  Port=7
  t_Hold_Position : Inport  Port=8
  CyclicTime : Inport  Port=9
  Saturation : Saturate  UpperLimit=150  LowerLimit=-150
  Saturation1 : Saturate  UpperLimit=500  LowerLimit=0
  Saturation2 : Saturate  UpperLimit=150  LowerLimit=0
  Saturation3 : Saturate  UpperLimit=500  LowerLimit=0
  Switch : Switch  Criteria=u2 > Threshold
  Switch1 : Switch  Criteria=u2 > Threshold
  WaveSignal : MATLAB Function  TreatAsAtomicUnit=on
  Position_Ref : Outport  VectorParamsAs1DForOutWhenUnconnected=off
  Velocity_Ref : Outport  Port=2  VectorParamsAs1DForOutWhenUnconnected=off
  acc_ref : Outport  Port=3  VectorParamsAs1DForOutWhenUnconnected=off
  Motion_Cycle_Time : Outport  Port=4  VectorParamsAs1DForOutWhenUnconnected=off
  Error : Outport  Port=5  VectorParamsAs1DForOutWhenUnconnected=off
  wires:
  CyclicTime/1 -> WaveSignal/8(t)
  WaveSignal/2(v) -> Switch/1
  Switch/1 -> Saturation/1
  v0/1 -> Switch/3, WaveSignal/2(v0)
  t0/1 -> WaveSignal/5(t0)
  Position_SP/1 -> Saturation3/1
  t_Hold_Position/1 -> WaveSignal/7(tWait)
  Velocity_SP/1 -> Saturation2/1
  WaveSignal/1(x) -> Switch1/1
  WaveSignal/4(T) -> Motion_Cycle_Time/1
  Enable/1 -> Switch1/2, Switch/2
  x0/1 -> Switch1/3, WaveSignal/1(x0)
  Switch1/1 -> Saturation1/1
  Saturation/1 -> Velocity_Ref/1
  Saturation1/1 -> Position_Ref/1
  WaveSignal/5(Error) -> Error/1
  Saturation2/1 -> WaveSignal/4(v_ref)
  Saturation3/1 -> WaveSignal/3(x_ref)
  t1/1 -> WaveSignal/6(tRamp)
  WaveSignal/3(a) -> acc_ref/1

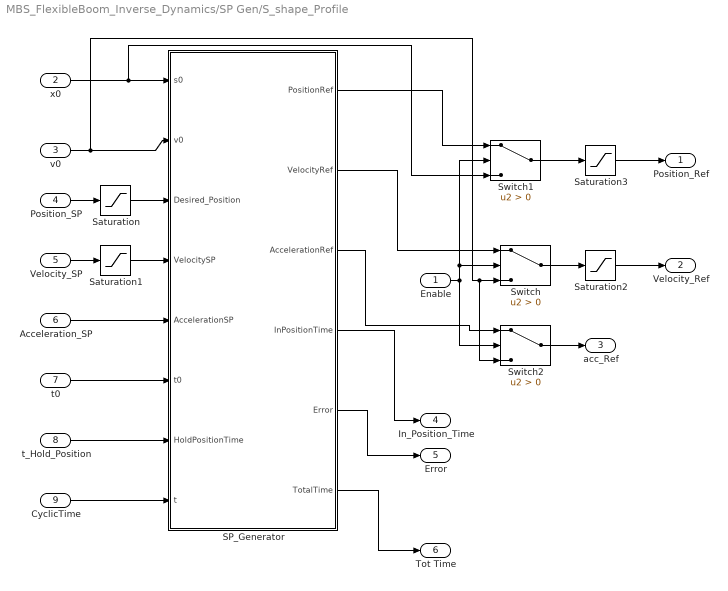
== system MBS_FlexibleBoom_Inverse_Dynamics/SP Gen/S_shape_Profile ==
  Enable : Inport  OutDataTypeStr=boolean
  x0 : Inport  Port=2
  v0 : Inport  Port=3
  Position_SP : Inport  Port=4
  Velocity_SP : Inport  Port=5
  Acceleration_SP : Inport  Port=6
  t0 : Inport  Port=7
  t_Hold_Position : Inport  Port=8
  CyclicTime : Inport  Port=9
  SP_Generator : MATLAB Function  TreatAsAtomicUnit=on
  Saturation : Saturate  UpperLimit=500  LowerLimit=0
  Saturation1 : Saturate  UpperLimit=150  LowerLimit=-150
  Saturation2 : Saturate  UpperLimit=150  LowerLimit=-150
  Saturation3 : Saturate  UpperLimit=500  LowerLimit=0
  Switch : Switch  Criteria=u2 > Threshold
  Switch1 : Switch  Criteria=u2 > Threshold
  Switch2 : Switch  Criteria=u2 > Threshold
  Position_Ref : Outport  VectorParamsAs1DForOutWhenUnconnected=off
  Velocity_Ref : Outport  Port=2  VectorParamsAs1DForOutWhenUnconnected=off
  acc_Ref : Outport  Port=3  VectorParamsAs1DForOutWhenUnconnected=off
  " In_Position_Time" : Outport  Port=4  VectorParamsAs1DForOutWhenUnconnected=off
  Error : Outport  Port=5  VectorParamsAs1DForOutWhenUnconnected=off
  Tot Time : Outport  Port=6  VectorParamsAs1DForOutWhenUnconnected=off
  wires:
  Saturation/1 -> SP_Generator/3(Desired_Position)
  Saturation1/1 -> SP_Generator/4(VelocitySP)
  t0/1 -> SP_Generator/6(t0)
  t_Hold_Position/1 -> SP_Generator/7(HoldPositionTime)
  Velocity_SP/1 -> Saturation1/1
  SP_Generator/4(InPositionTime) -> " In_Position_Time"/1
  CyclicTime/1 -> SP_Generator/8(t)
  SP_Generator/5(Error) -> Error/1
  Position_SP/1 -> Saturation/1
  Saturation2/1 -> Velocity_Ref/1
  Switch/1 -> Saturation2/1
  x0/1 -> Switch1/3, SP_Generator/1(s0)
  SP_Generator/1(PositionRef) -> Switch1/1
  Saturation3/1 -> Position_Ref/1
  Enable/1 -> Switch2/2, Switch1/2, Switch/2
  SP_Generator/2(VelocityRef) -> Switch/1
  Switch1/1 -> Saturation3/1
  SP_Generator/6(TotalTime) -> Tot Time/1
  Acceleration_SP/1 -> SP_Generator/5(AccelerationSP)
  v0/1 -> Switch2/3, Switch/3, SP_Generator/2(v0)
  SP_Generator/3(AccelerationRef) -> Switch2/1
  Switch2/1 -> acc_Ref/1
